simulink model "hydraulic_pilot_SimMechanics_end_US"  (R2015b)
settings: Solver=ode23t  StartTime=0.0  StopTime=1500  RelTol=1e-3
undefined symbols (not defined in the file): sigbuilder_block, X, Y, Z
libraries: sm_lib x295, fl_lib x24, nesl_utility x11, sh_lib x5, simulink x1
(part 1 of 7)
settings Model: Creator=Ivan  LastModifiedBy=Ivan
settings DataIOCC: SaveFormat=Array
settings DebuggingCC: UnderspecifiedInitializationDetection=Classic  MergeDetectMultiDrivingBlocksExec=none  SolverPrmCheckMsg=warning  StateNameClashWarn=warning
settings HardwareCC: ProdBitPerPointer=32  ProdLargestAtomicFloat=None  ProdIntDivRoundTo=Undefined  ProdEndianess=Unspecified  ProdWordSize=32  ProdHWDeviceType=32-bit Generic
settings GRTTargetCC: GeneratePreprocessorConditionals=Disable all
settings ConfigComp: CovModelRefEnable=Off
settings SimscapeCC: SimscapeLogType=all  SimscapeLogLimitData=off
settings ExplorerConfigSet: InternalSimMechanicsExplorerSettings="<ExplorerConfiguration><canonicalview>default</canonicalview><AnimationSetting><BasePlaybackSpeed>1.0</BasePlaybackSpeed><PlaybackSpeedFactor>16.0</PlaybackSpeedFactor></AnimationSetting><TilePanel><TileInfo><Tiles Columns=\"2\" Count=\"4\" Rows=\"2\"><Column Left=\"2\" Weight=\"0.5\"/><Column Left=\"554\" Weight=\"0.5\"/><Column Left=\"1106\"/><Row Top=\"2\" Weight=\"0.4992\"/><Row Top=\"320\" Weight=\"0.5008\"/><Row Top=\"639\"/><Tile Height=\"1\" Width=\"1\" X=\"0\" Y=\"0\"/><Tile Height=\"1\" Width=\"1\" X=\"0\" Y=\"1\"/><Tile Height=\"1\" Width=\"1\" X=\"1\" Y=\"0\"/><Tile Height=\"1\" Width=\"1\" X=\"1\" Y=\"1\"/></Tiles></TileInfo><SceneInfo><SceneViewer><BGColor><R>0.60000002384185791</R><G>0.60000002384185791</G><B>0.60000002384185791</B></BGColor><Camera><Position><X>-1.4545420789578025</X><Y>-0.47703526853152423</Y><Z>1.053292472596125</Z></Position><Center><X>-1.0755331343287176</X><Y>0.65681441625729753</Y><Z>0.33046154790126991</Z></Center><Up><X>0.31799715127972389</X><Y>0.43179203595848165</Y><Z>0.84405772874893448</Z></Up><Left>-0.52137946486473086</Left><Right>0.52137946486473086</Right><Bottom>-0.12744375988841058</Bottom><Top>0.12744375988841058</Top></Camera></SceneViewer><SceneViewer><BGColor><R>0.60000002384185791</R><G>0.60000002384185791</G><B>0.60000002384185791</B></BGColor><Camera><Position><X>-1.097124655307177</X><Y>0.60879350298107193</Y><Z>1.6773847746848054</Z></Position><Center><X>-1.097124655307177</X><Y>0.60879350298107193</Y><Z>0.3230140209197998</Z></Center><Up><X>0</X><Y>1</Y><Z>-0</Z></Up><Left>-0.52137946486473086</Left><Right>0.52137946486473086</Right><Bottom>-0.19162502065300943</Bottom><Top>0.19162502065300943</Top></Camera></SceneViewer><SceneViewer><BGColor><R>0.60000002384185791</R><G>0.60000002384185791</G><B>0.60000002384185791</B></BGColor><Camera><Position><X>-1.839713975613805</X><Y>1.4497817237667032</Y><Z>1.0667372871108483</Z></Position><Center><X>-1.0007040048852538</X><Y>0.55541256489420043</Y><Z>0.26430212739881542</Z></Center><Up><X>0.29701754457873719</X><Y>-0.46808723288325788</Y><Z>0.83227094183571793</Z></Up><Left>-0.47525307471029621</Left><Right>0.47525307471029621</Right><Bottom>-0.31607583672115108</Bottom><Top>0.31607583672115108</Top></Camera></SceneViewer><SceneViewer><BGColor><R>0.60000002384185791</R><G>0.60000002384185791</G><B>0.60000002384185791</B></BGColor><Camera><Position><X>-0.30663977538297038</X><Y>-0.17371608341982503</Y><Z>1.1012231263046517</Z></Position><Center><X>-1.0848488807678223</X><Y>0.60449302196502686</Y><Z>0.3230140209197998</Z></Center><Up><X>-0.40824829046386307</X><Y>0.40824829046386307</Y><Z>0.81649658092772615</Z></Up><Left>-0.50417031347751617</Left><Right>0.50417031347751617</Right><Bottom>-0.39514026045799255</Bottom><Top>0.39514026045799255</Top></Camera></SceneViewer></SceneInfo></TilePanel></ExplorerConfiguration>"

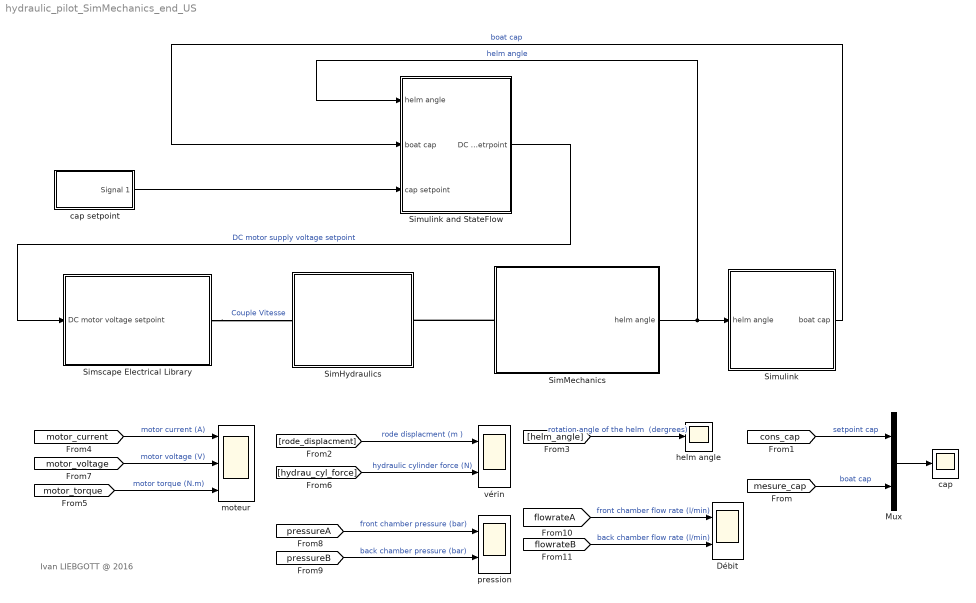
== system hydraulic_pilot_SimMechanics_end_US ==
  note: Ivan LIEBGOTT @ 2016
  " moteur" : Scope  NumInputPorts=3
  Débit : Scope  NumInputPorts=2
  Mux : Mux  Inputs=2
  SimHydraulics : Subsystem
      mask Display: image('groupe_hydraulique.jpg')
  SimMechanics : Subsystem
      mask Display: image('pilote_simmechanics.jpg')
  "Simscape Electrical Library " : Subsystem
      mask Display: image('moteur_cc_pilote.jpg')
  Simulink : Subsystem
      mask Display: image('bateau.jpg')
  Simulink and StateFlow : Subsystem
      mask Display: image('AP16_FRONT.jpg')
  "cap " : Scope
  cap setpoint : Subsystem  Tag=STV Subsys  LoadFcn=sigbuilder_block('load');  StartFcn=sigbuilder_block('start');  StopFcn=sigbuilder_block('stop');  ClipboardFcn=sigbuilder_block('clipboard');  mask(Sigbuilder block){}
      mask help: Simulink:masks:SigbuilderBlock_MD
      mask init:
      | if ~strcmp(get_param(bdroot(gcbh),'SimulationStatus'),'stopped') tuvar = sigbuilder_block('maskInit'); end
      settings: CopyFcn=sigbuilder_block('copy');  DeleteFcn=sigbuilder_block('delete');  ModelCloseFcn=sigbuilder_block('modelClose');  PreSaveFcn=sigbuilder_block('preSave');  PauseFcn=sigbuilder_block('pause');  ContinueFcn=sigbuilder_block('continue');  NameChangeFcn=sigbuilder_block('namechange');  OpenFcn=sigbuilder_block('open',[286.5 145 550.5 396 ]);  CloseFcn=sigbuilder_block('close');
      mask Display: plot(0, 0, 100, 100,[2, 2, 32, 32, 2], [68, 8, 8, 68, 68],[32, 2], [38, 38], [32, 19, 2],[53, 60, 44], [32, 17, 17, 2],[16, 16, 31, 31]);txt = getActiveGroup(gcbh);text(2, 100, txt,'verticalAlignment', 'top');
  helm angle : Scope
  pression : Scope  NumInputPorts=2
  vérin : Scope  NumInputPorts=2
  wires:
  Mux/1 -> "cap "/1
  [mesure_cap] -> Mux/2  "boat cap"
  [cons_cap] -> Mux/1  "setpoint cap"
  [rode_displacment] -> vérin/1  "rode displacment (m )"
  [helm_angle] -> helm angle/1  "rotation angle of the helm  (dergrees)"
  [motor_current] -> " moteur"/1  "motor current (A)"
  [motor_torque] -> " moteur"/3  "motor torque (N.m)"
  [hydrau_cyl_force] -> vérin/2  "hydraulic cylinder force (N)"
  cap setpoint/1(Signal 1) -> Simulink and StateFlow/3(cap setpoint)
  Simulink/1(boat cap) -> Simulink and StateFlow/2(boat cap)  "boat cap"
  Simulink and StateFlow/1(DC motor voltage setrpoint) -> "Simscape Electrical Library "/1(DC motor voltage setpoint)  "DC motor supply voltage setpoint"
  [motor_voltage] -> " moteur"/2  "motor voltage (V)"
  [pressureA] -> pression/1  "front chamber pressure (bar)"
  [pressureB] -> pression/2  "back chamber pressure (bar)"
  [flowrateA] -> Débit/1  "front chamber flow rate (l/min)"
  [flowrateB] -> Débit/2  "back chamber flow rate (l/min)"
  SimMechanics/1(helm angle) -> Simulink and StateFlow/1(helm angle), Simulink/1(helm angle)  "helm angle"
  connections:
  "Simscape Electrical Library "/RConn1 -- SimHydraulics/LConn1  "Couple Vitesse"
  SimMechanics/LConn1 -- SimHydraulics/RConn1

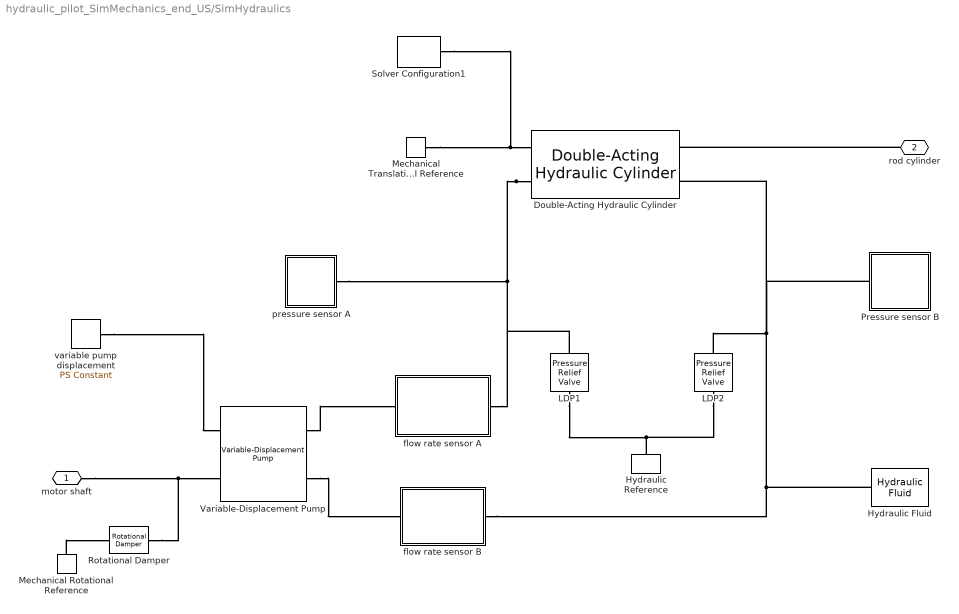
== system hydraulic_pilot_SimMechanics_end_US/SimHydraulics ==
  " LDP1" : sh_lib/Valves/Pressure Control Valves/Pressure Relief Valve  area_max=1e-4 m^2  pres_set=10e+6 Pa  reg_range=5e+5 Pa  C_d=0.7  Re_cr=12  A_leak=1e-12 m^2  dynamic=0  tau=0.1 s  area_init=1e-12 m^2  gain=1 m^2/Pa  pr_max=55e5 Pa  f_cr=100 N
  Double-Acting Hydraulic Cylinder : sh_lib/Hydraulic Cylinders/Double-Acting Hydraulic Cylinder  area_A=2e-4 m^2  area_B=2e-4 m^2  stroke=0.3 m  init_pos=0.15 m  dead_vol_A=1e-4 m^3  dead_vol_B=1e-4 m^3  init_pressure_A=0 Pa  init_pressure_B=0 Pa  k_sh=1.4  stiff=1e+6 N/m  D=150 N/(m/s)  or=1  or_sign=1
  Hydraulic Fluid : sh_lib/Hydraulic Utilities/Hydraulic Fluid  DataSource=1  SelFluid=1  SysTemp=60 c  TrapAir=0.005  ViscDerFactor=1  range_error=2
  Hydraulic Reference : fl_lib/Hydraulic/Hydraulic Elements/Hydraulic Reference
  LDP2 : sh_lib/Valves/Pressure Control Valves/Pressure Relief Valve  area_max=1e-4 m^2  pres_set=10e+6 Pa  reg_range=5e+5 Pa  C_d=0.7  Re_cr=12  A_leak=1e-12 m^2  dynamic=0  tau=0.1 s  area_init=1e-12 m^2  gain=1 m^2/Pa  pr_max=55e5 Pa  f_cr=100 N
  Mechanical Rotational Reference : fl_lib/Mechanical/Rotational Elements/Mechanical Rotational Reference
  Mechanical Translational Reference : fl_lib/Mechanical/Translational Elements/Mechanical Translational Reference
  Pressure sensor B : Subsystem
      mask Display: image('manometre.jpg')
  Rotational Damper : fl_lib/Mechanical/Rotational Elements/Rotational Damper  D=0.006 N*m/(rad/s)  w_specify=off  w_priority=None  w=0 rad/s  t_specify=off  t_priority=None  t=0 N*m
  Solver Configuration1 : nesl_utility/Solver Configuration  PhysicalDomain=network_engine_domain  SubClassName=solver  LeftPortType=input  RightPortType=generic  Accelerate=off  Tones=[]  Harmonics=[]  SimulateNoise=off  Profile=off  UseLocalSampling=off  EnableSwitchedLinearOptims=on  FrequencyDomain=off  UseCCode=off  RelTol=0.001  AbsTol=1e-06  MinStep=1e-09  ToWorkspace=off  RevertToSquareIcSolve=off  NumHomotopyIterations=100  PhasorMode=off  PhasorModeNumHarmonics=1  DoDC=off  ResidualTolerance=1e-09  UseLocalSolver=off  LocalSolverChoice=NE_BACKWARD_EULER_ADVANCER  LocalSolverSampleTime=0.001  DoFixedCost=off  MaxNonlinIter=3  MaxModeIter=2  LinearAlgebra=Sparse  DelaysMemoryBudget=1024  AutomaticFiltering=on  FilteringTimeConstant=0.001
  Variable-Displacement Pump : sh_lib/Pumps and Motors/Variable-Displacement Pump  mdl_type=1  D_max=1.77e-7 m^3/rad  stroke_max=1 m  displ_tab=[ -5e-6 -3e-6 0 3e-6 5e-6 ] m^3/rad  cntrl_mem_tab=[ -0.0075 -0.0025 0 0.0025 0.0075 ] m  interp_method=1  extrap_method=1  efficiency_vol=0.85  efficiency_tot=0.75  pr_nominal=1e+8 Pa  w_nominal=188 rad/s  visc_nominal=18 cSt  dens_nominal=900 kg/m^3  k_leak=1e-11 m^3/s/Pa  efficiency_mech=0.7
  flow rate sensor A : Subsystem
      mask Display: image('debimetre.jpg')
  flow rate sensor B : Subsystem
      mask Display: image('debimetre.jpg')
  pressure sensor A : Subsystem
      mask Display: image('manometre.jpg')
  variable pump displacement : fl_lib/Physical Signals/Sources/PS Constant  constant=0.4
  motor shaft : PMIOPort  Port=1  Side=Left
  rod cylinder : PMIOPort  Port=2  Side=Right
  connections:
  motor shaft/RConn1 -- Rotational Damper/RConn1 -- Variable-Displacement Pump/LConn2
  variable pump displacement/RConn1 -- Variable-Displacement Pump/LConn1
  rod cylinder/RConn1 -- Double-Acting Hydraulic Cylinder/RConn1
  Mechanical Translational Reference/LConn1 -- Solver Configuration1/RConn1 -- Double-Acting Hydraulic Cylinder/LConn1
  Hydraulic Fluid/RConn1 -- flow rate sensor B/RConn1 -- Pressure sensor B/LConn1 -- Double-Acting Hydraulic Cylinder/RConn2 -- LDP2/LConn1
  Hydraulic Reference/LConn1 -- " LDP1"/RConn1 -- LDP2/RConn1
  Mechanical Rotational Reference/LConn1 -- Rotational Damper/LConn1
  Double-Acting Hydraulic Cylinder/LConn2 -- flow rate sensor A/RConn1 -- " LDP1"/LConn1 -- pressure sensor A/RConn1
  Variable-Displacement Pump/RConn1 -- flow rate sensor A/LConn1
  Variable-Displacement Pump/RConn2 -- flow rate sensor B/LConn1

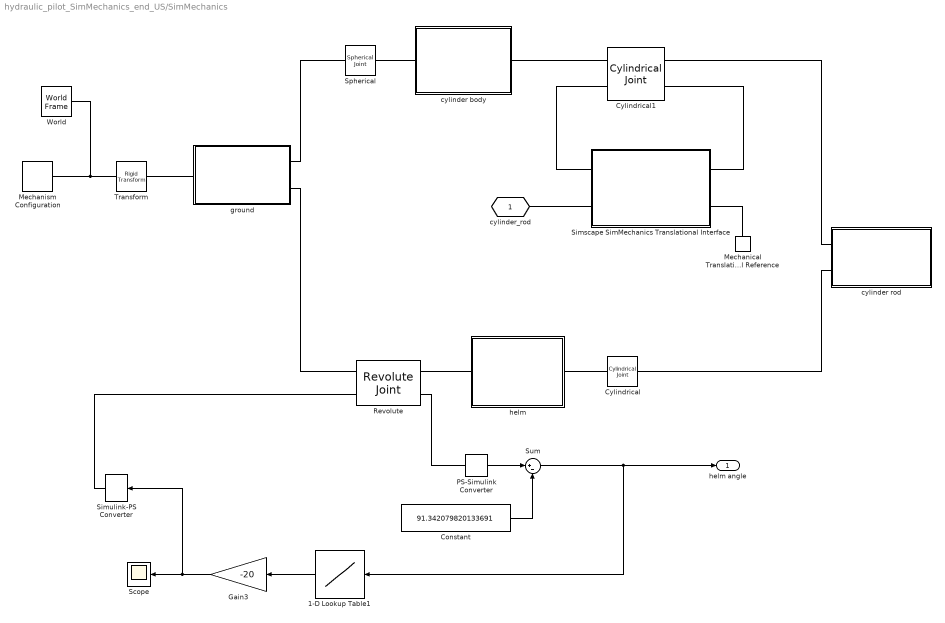
== system hydraulic_pilot_SimMechanics_end_US/SimMechanics ==
  1-D Lookup Table1 : Lookup_n-D  NumberOfTableDimensions=1  BreakpointsForDimension1=[0 5 10 15 20 25 30]  Table=[0 2.5 5 10 30 60 100]  RndMeth=Simplest  InputSameDT=on
  Constant : Constant  Value=91.342079820133691
  Cylindrical : sm_lib/Joints/Cylindrical Joint  SenseConstraintForce=off  SenseConstraintForceX=off  SenseConstraintForceY=off  SenseConstraintForceZ=off  SenseConstraintTorque=off  SenseConstraintTorqueX=off  SenseConstraintTorqueY=off  SenseConstraintTorqueZ=off  SenseTotalForce=off  SenseTotalForceX=off  SenseTotalForceY=off  SenseTotalForceZ=off  SenseTotalTorque=off  SenseTotalTorqueX=off  SenseTotalTorqueY=off  SenseTotalTorqueZ=off  CompositeWrenchDir=FollowerOnBase  CompositeWrenchFrame=BaseFrame  PzEquilibriumPosition=0  PzEquilibriumPositionUnits=m  PzSpringStiffness=0  PzSpringStiffnessUnits=N/m  PzDampingCoefficient=0  PzDampingCoefficientUnits=s*N/m  PzTorqueActuationMode=NoTorque  PzMotionActuationMode=ComputedMotion  PzSensePosition=off  PzSenseVelocity=off  PzSenseAcceleration=off  PzSenseTorqueForce=off  PzPositionTargetSpecify=on  PzPositionTargetPriority=Low  PzPositionTargetValue=0  PzPositionTargetValueUnits=m  PzVelocityTargetSpecify=off  PzVelocityTargetPriority=High  PzVelocityTargetValue=0  PzVelocityTargetValueUnits=m/s  RzEquilibriumPosition=0  RzEquilibriumPositionUnits=rad  RzSpringStiffness=0  RzSpringStiffnessUnits=m*N/rad  RzDampingCoefficient=0  RzDampingCoefficientUnits=m*s*N/rad  RzTorqueActuationMode=NoTorque  RzMotionActuationMode=ComputedMotion  RzSensePosition=off  RzSenseVelocity=off  RzSenseAcceleration=off  RzSenseTorqueForce=off  RzPositionTargetSpecify=on  RzPositionTargetPriority=Low  RzPositionTargetValue=88.917590363493801  RzPositionTargetValueUnits=deg  RzVelocityTargetSpecify=off  RzVelocityTargetPriority=High  RzVelocityTargetValue=0  RzVelocityTargetValueUnits=deg/s  BlockFunction=simmechanics.library.joints.cylindrical_joint
  Cylindrical1 : sm_lib/Joints/Cylindrical Joint  SenseConstraintForce=off  SenseConstraintForceX=off  SenseConstraintForceY=off  SenseConstraintForceZ=off  SenseConstraintTorque=off  SenseConstraintTorqueX=off  SenseConstraintTorqueY=off  SenseConstraintTorqueZ=off  SenseTotalForce=off  SenseTotalForceX=off  SenseTotalForceY=off  SenseTotalForceZ=off  SenseTotalTorque=off  SenseTotalTorqueX=off  SenseTotalTorqueY=off  SenseTotalTorqueZ=off  CompositeWrenchDir=FollowerOnBase  CompositeWrenchFrame=BaseFrame  PzEquilibriumPosition=0  PzEquilibriumPositionUnits=m  PzSpringStiffness=0  PzSpringStiffnessUnits=N/m  PzDampingCoefficient=200  PzDampingCoefficientUnits=s*N/m  PzTorqueActuationMode=InputTorque  PzMotionActuationMode=ComputedMotion  PzSensePosition=off  PzSenseVelocity=on  PzSenseAcceleration=off  PzSenseTorqueForce=off  PzPositionTargetSpecify=on  PzPositionTargetPriority=Low  PzPositionTargetValue=0  PzPositionTargetValueUnits=m  PzVelocityTargetSpecify=off  PzVelocityTargetPriority=High  PzVelocityTargetValue=0  PzVelocityTargetValueUnits=m/s  RzEquilibriumPosition=0  RzEquilibriumPositionUnits=rad  RzSpringStiffness=0  RzSpringStiffnessUnits=m*N/rad  RzDampingCoefficient=1  RzDampingCoefficientUnits=m*s*N/rad  RzTorqueActuationMode=NoTorque  RzMotionActuationMode=ComputedMotion  RzSensePosition=off  RzSenseVelocity=off  RzSenseAcceleration=off  RzSenseTorqueForce=off  RzPositionTargetSpecify=on  RzPositionTargetPriority=Low  RzPositionTargetValue=-151.66852375213551  RzPositionTargetValueUnits=deg  RzVelocityTargetSpecify=off  RzVelocityTargetPriority=High  RzVelocityTargetValue=0  RzVelocityTargetValueUnits=deg/s  BlockFunction=simmechanics.library.joints.cylindrical_joint
  Gain3 : Gain  Gain=-20
  Mechanical Translational Reference : fl_lib/Mechanical/Translational Elements/Mechanical Translational Reference
  Mechanism Configuration : sm_lib/Utilities/Mechanism Configuration  UniformGravity=Constant  GravityVector=[0 0 -9.81]  GravityUnits=m/s^2  LinearizationDelta=0.001  BlockFunction=simmechanics.library.utilities.mechanism_configuration
  PS-Simulink Converter : nesl_utility/PS-Simulink Converter  PhysicalDomain=network_engine_domain  SubClassName=ps_output  LeftPortType=input  RightPortType=output  PseudoPeriodic=off  Frequencies=[]  Unit=deg  AffineConversion=off
  Revolute : sm_lib/Joints/Revolute Joint  SenseConstraintForce=off  SenseConstraintForceX=off  SenseConstraintForceY=off  SenseConstraintForceZ=off  SenseConstraintTorque=off  SenseConstraintTorqueX=off  SenseConstraintTorqueY=off  SenseConstraintTorqueZ=off  SenseTotalForce=off  SenseTotalForceX=off  SenseTotalForceY=off  SenseTotalForceZ=off  SenseTotalTorque=off  SenseTotalTorqueX=off  SenseTotalTorqueY=off  SenseTotalTorqueZ=off  CompositeWrenchDir=FollowerOnBase  CompositeWrenchFrame=BaseFrame  EquilibriumPosition=0  EquilibriumPositionUnits=rad  SpringStiffness=0  SpringStiffnessUnits=m*N/rad  DampingCoefficient=0  DampingCoefficientUnits=m*s*N/rad  TorqueActuationMode=InputTorque  MotionActuationMode=ComputedMotion  SensePosition=on  SenseVelocity=off  SenseAcceleration=off  SenseTorqueForce=off  PositionTargetSpecify=on  PositionTargetPriority=Low  PositionTargetValue=91.342079820133691  PositionTargetValueUnits=deg  VelocityTargetSpecify=off  VelocityTargetPriority=High  VelocityTargetValue=0  VelocityTargetValueUnits=deg/s  BlockFunction=simmechanics.library.joints.revolute_joint
  Scope : Scope
  Simscape SimMechanics Translational Interface : Subsystem
  Simulink-PS Converter : nesl_utility/Simulink-PS Converter  PhysicalDomain=network_engine_domain  SubClassName=ps_input  LeftPortType=input  RightPortType=output  PseudoPeriodic=off  Frequencies=[]  NoiseDistribution=none  NoiseParameters=[]  Unit=1  AffineConversion=off  InputFiltering=off  SimscapeFilterOrder=1  InputFilterTimeConstant=0.001  UdotUserProvided=1
  Spherical : sm_lib/Joints/Spherical Joint  SenseConstraintForce=off  SenseConstraintForceX=off  SenseConstraintForceY=off  SenseConstraintForceZ=off  SenseConstraintTorque=off  SenseConstraintTorqueX=off  SenseConstraintTorqueY=off  SenseConstraintTorqueZ=off  SenseTotalForce=off  SenseTotalForceX=off  SenseTotalForceY=off  SenseTotalForceZ=off  SenseTotalTorque=off  SenseTotalTorqueX=off  SenseTotalTorqueY=off  SenseTotalTorqueZ=off  CompositeWrenchDir=FollowerOnBase  CompositeWrenchFrame=BaseFrame  DefPosRotationMethod=None  DefPosRotationAngleUnits=deg  DefPosRotationStandardAxis=+Z  DefPosRotationAngle=0  DefPosRotationArbitraryAxis=[0 0 1]  DefPosFollAlignAxisA=+X  DefPosBaseAlignAxisA=+Y  DefPosFollAlignAxisB=+Y  DefPosBaseAlignAxisB=+Z  DefPosRotationSequenceAxes=FollowerAxes  DefPosRotationSequence=XYX  DefPosRotationSequenceAngles=[0 0 0]  DefPosRotationSequenceAnglesUnits=deg  DefPosRotationMatrix=[1 0 0; 0 1 0; 0 0 1]  EqPosRotationMethod=None  EqPosRotationAngleUnits=deg  EqPosRotationStandardAxis=+Z  EqPosRotationAngle=0  EqPosRotationArbitraryAxis=[0 0 1]  EqPosFollAlignAxisA=+X  EqPosBaseAlignAxisA=+Y  EqPosFollAlignAxisB=+Y  EqPosBaseAlignAxisB=+Z  EqPosRotationSequenceAxes=FollowerAxes  EqPosRotationSequence=XYX  EqPosRotationSequenceAngles=[0 0 0]  EqPosRotationSequenceAnglesUnits=deg  EqPosRotationMatrix=[1 0 0; 0 1 0; 0 0 1]  SpringStiffness=0  SpringStiffnessUnits=m*N/rad  DampingCoefficient=0  DampingCoefficientUnits=m*s*N/rad  ActuateTorqueX=off  ActuateTorqueY=off  ActuateTorqueZ=off  ActuateTorque=off  TorqueActuationMode=NoTorque  MotionActuationMode=ComputedMotion  ActuationFrame=BaseFrame  SensePosition=off  SenseVelocityX=off  SenseVelocityY=off  SenseVelocityZ=off  SenseVelocity=off  SenseAccelerationX=off  SenseAccelerationY=off  SenseAccelerationZ=off  SenseAcceleration=off  SenseTorqueX=off  SenseTorqueY=off  SenseTorqueZ=off  SenseTorqueForce=off  SensingFrame=FollowerFrame  PositionTargetRotationMethod=None  PositionTargetRotationAngleUnits=deg  PositionTargetRotationStandardAxis=+Z  PositionTargetRotationAngle=0  PositionTargetRotationArbitraryAxis=[0 0 1]  PositionTargetFollAlignAxisA=+X  PositionTargetBaseAlignAxisA=+Y  PositionTargetFollAlignAxisB=+Y  PositionTargetBaseAlignAxisB=+Z  PositionTargetRotationSequenceAxes=FollowerAxes  PositionTargetRotationSequence=XYX  PositionTargetRotationSequenceAngles=[0 0 0]  PositionTargetRotationSequenceAnglesUnits=deg  PositionTargetRotationMatrix=[1 0 0; 0 1 0; 0 0 1]  PositionTargetSpecify=off  PositionTargetPriority=High  VelocityTargetValue=[0 0 0]  VelocityTargetValueUnits=deg/s  VelocityTargetSpecify=off  VelocityTargetPriority=High  VelocityTargetInFollowerFrame=on  BlockFunction=simmechanics.library.joints.spherical_joint
  Sum : Sum  Inputs=|+-
  Transform : sm_lib/Frames and Transforms/Rigid Transform  TranslationMethod=Cartesian  TranslationLengthUnit=mm  TranslationStandardAxis=+Z  TranslationStandardOffset=0  TranslationCartesianOffset=[-854.29700000000003 517.99300000000005 336.38900000000001]  TranslationROffset=0  TranslationROffsetUnits=m  TranslationZOffset=0  TranslationZOffsetUnits=m  TranslationThetaOffset=0  TranslationThetaOffsetUnits=deg  RotationMethod=None  RotationAngleUnits=deg  RotationStandardAxis=+Z  RotationAngle=0  RotationArbitraryAxis=[0 0 1]  FollAlignAxisA=+X  BaseAlignAxisA=+Y  FollAlignAxisB=+Y  BaseAlignAxisB=+Z  RotationSequenceAxes=FollowerAxes  RotationSequence=XYX  RotationSequenceAngles=[0 0 0]  RotationSequenceAnglesUnits=deg  RotationMatrix=[1 0 0; 0 1 0; 0 0 1]  BlockFunction=simmechanics.library.frames_transforms.rigid_transform
  World : sm_lib/Frames and Transforms/World Frame  BlockFunction=simmechanics.library.frames_transforms.world_frame
  cylinder body : Subsystem
      mask Display: image('cylindre.jpg')
  cylinder rod : Subsystem
      mask Display: image('tige1.jpg')
  ground : Subsystem
      mask Display: image('bati1.jpg')
  helm : Subsystem
      mask Display: image('meche.jpg')
  "cylinder_rod " : PMIOPort  Port=1  Side=Left
  helm angle : Outport
  wires:
  Constant/1 -> Sum/2
  Sum/1 -> 1-D Lookup Table1/1, helm angle/1
  1-D Lookup Table1/1 -> Gain3/1
  Gain3/1 -> Simulink-PS Converter/1, Scope/1
  PS-Simulink Converter/1 -> Sum/1
  connections:
  World/RConn1 -- Transform/LConn1 -- Mechanism Configuration/RConn1
  Revolute/RConn1 -- helm/LConn1
  cylinder body/LConn1 -- Spherical/RConn1
  Cylindrical1/RConn1 -- cylinder rod/LConn1
  Cylindrical/LConn1 -- helm/RConn1
  Cylindrical/RConn1 -- cylinder rod/LConn2
  ground/RConn1 -- Spherical/LConn1
  ground/LConn1 -- Transform/RConn1
  Revolute/LConn1 -- ground/RConn2
  Cylindrical1/LConn1 -- cylinder body/RConn1
  Cylindrical1/RConn2 -- Simscape SimMechanics Translational Interface/RConn1
  Mechanical Translational Reference/LConn1 -- Simscape SimMechanics Translational Interface/RConn2
  "cylinder_rod "/RConn1 -- Simscape SimMechanics Translational Interface/LConn2
  Simscape SimMechanics Translational Interface/LConn1 -- Cylindrical1/LConn2
  Revolute/RConn2 -- PS-Simulink Converter/LConn1
  Simulink-PS Converter/RConn1 -- Revolute/LConn2

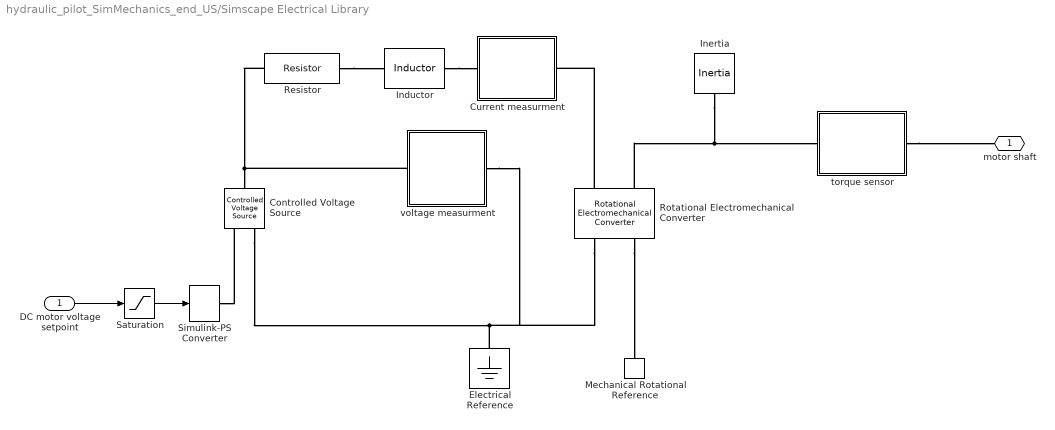
== system hydraulic_pilot_SimMechanics_end_US/Simscape Electrical Library  ==
  DC motor voltage setpoint : Inport
  Controlled Voltage Source : fl_lib/Electrical/Electrical Sources/Controlled Voltage Source
  Current measurment : Subsystem
      mask Display: image('ampermetre.jpg')
  Electrical Reference : fl_lib/Electrical/Electrical Elements/Electrical Reference
  Inductor : fl_lib/Electrical/Electrical Elements/Inductor  l=1e-7 H  r=0 Ohm  g=1e-9 1/Ohm  i_specify=off  i_priority=None  i=0 A  v_specify=off  v_priority=None  v=0 V  i_L_specify=on  i_L_priority=High  i_L=0 A
  Inertia : fl_lib/Mechanical/Rotational Elements/Inertia  inertia=0.005 kg*m^2  w_specify=on  w_priority=High  w=0 rad/s  t_specify=off  t_priority=None  t=0 N*m
  Mechanical Rotational Reference : fl_lib/Mechanical/Rotational Elements/Mechanical Rotational Reference
  Resistor : fl_lib/Electrical/Electrical Elements/Resistor  R=0.247 Ohm  i_specify=off  i_priority=None  i=0 A  v_specify=off  v_priority=None  v=0 V
  Rotational Electromechanical Converter : fl_lib/Electrical/Electrical Elements/Rotational Electromechanical Converter  K=0.047 V/(rad/s)  i_specify=off  i_priority=None  i=0 A  v_specify=off  v_priority=None  v=0 V  t_specify=off  t_priority=None  t=0 N*m  w_specify=off  w_priority=None  w=0 rad/s
  Saturation : Saturate  UpperLimit=12  LowerLimit=-12
  Simulink-PS Converter : nesl_utility/Simulink-PS Converter  PhysicalDomain=network_engine_domain  SubClassName=ps_input  LeftPortType=input  RightPortType=output  PseudoPeriodic=off  Frequencies=[]  NoiseDistribution=none  NoiseParameters=[]  Unit=V  AffineConversion=off  InputFiltering=off  SimscapeFilterOrder=1  InputFilterTimeConstant=0.001  UdotUserProvided=1
  torque sensor : Subsystem
      mask Display: image('couplemetre.jpg')
  voltage measurment : Subsystem
      mask Display: image('voltmetre.jpg')
  motor shaft : PMIOPort  Port=1  Side=Right
  wires:
  DC motor voltage setpoint/1 -> Saturation/1
  Saturation/1 -> Simulink-PS Converter/1
  connections:
  Simulink-PS Converter/RConn1 -- Controlled Voltage Source/RConn1
  Rotational Electromechanical Converter/RConn2 -- Mechanical Rotational Reference/LConn1
  Electrical Reference/LConn1 -- Controlled Voltage Source/RConn2 -- voltage measurment/RConn1 -- Rotational Electromechanical Converter/RConn1
  Resistor/LConn1 -- voltage measurment/LConn1 -- Controlled Voltage Source/LConn1
  Resistor/RConn1 -- Inductor/LConn1
  Inductor/RConn1 -- Current measurment/LConn1
  Rotational Electromechanical Converter/LConn1 -- Current measurment/RConn1
  Inertia/LConn1 -- Rotational Electromechanical Converter/LConn2 -- torque sensor/LConn1
  torque sensor/RConn1 -- motor shaft/RConn1

== system hydraulic_pilot_SimMechanics_end_US/Simulink ==
  helm angle : Inport
  Integrator : Integrator
  Perturbation : Subsystem
      mask Display: image('vague.jpg')
  Sum : Sum  Inputs=-+|
  Transfer Fcn1 : TransferFcn  Numerator=[0.005]  Denominator=[1 0.1]
  boat cap : Outport
  wires:
  helm angle/1 -> Transfer Fcn1/1
  Integrator/1 -> boat cap/1
  Sum/1 -> Integrator/1
  Transfer Fcn1/1 -> Sum/2
  Perturbation/1(Out1) -> Sum/1

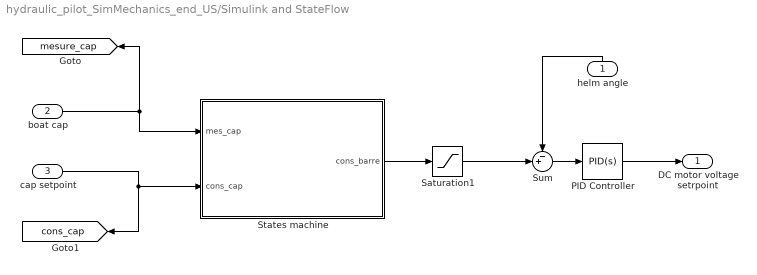
== system hydraulic_pilot_SimMechanics_end_US/Simulink and StateFlow ==
  helm angle : Inport
  boat cap : Inport  Port=2
  cap setpoint : Inport  Port=3
  PID Controller : simulink/Continuous/PID Controller  Controller=PID  TimeDomain=Continuous-time  SampleTime=-1  IntegratorMethod=Forward Euler  FilterMethod=Forward Euler  Form=Parallel  UseFilter=on  ControllerParametersSource=internal  P=0.5  I=0.001  D=0  N=100  InitialConditionSource=internal  InitialConditionForIntegrator=0  InitialConditionForFilter=0  ExternalReset=none  LimitOutput=off  UpperSaturationLimit=inf  LowerSaturationLimit=-inf  LinearizeAsGain=on  AntiWindupMode=none  Kb=1  TrackingMode=off  Kt=1  PParamMin=[]  PParamMax=[]  IParamMin=[]  IParamMax=[]  DParamMin=[]  DParamMax=[]  NParamMin=[]  NParamMax=[]  KbParamMin=[]  KbParamMax=[]  KtParamMin=[]  KtParamMax=[]  POutMin=[]  POutMax=[]  IOutMin=[]  IOutMax=[]  DOutMin=[]  DOutMax=[]  NOutMin=[]  NOutMax=[]  KbOutMin=[]  KbOutMax=[]  KtOutMin=[]  KtOutMax=[]  IntegratorOutMin=[]  IntegratorOutMax=[]  FilterOutMin=[]  FilterOutMax=[]  SumOutMin=[]  SumOutMax=[]  SumI1OutMin=[]  SumI1OutMax=[]  SumI2OutMin=[]  SumI2OutMax=[]  SumI3OutMin=[]  SumI3OutMax=[]  SumDOutMin=[]  SumDOutMax=[]  SaturationOutMin=[]  SaturationOutMax=[]  IntegratorContinuousStateAttributes=''  IntegratorStateMustResolveToSignalObject=off  IntegratorRTWStateStorageClass=Auto  FilterContinuousStateAttributes=''  FilterStateMustResolveToSignalObject=off  FilterRTWStateStorageClass=Auto  DifferentiatorICPrevScaledInput=0  DifferentiatorOutMin=[]  DifferentiatorOutMax=[]
  Saturation1 : Saturate  UpperLimit=25  LowerLimit=-25
  States machine : Stateflow chart  TreatAsAtomicUnit=on
  Sum : Sum  Inputs=-+|
  DC motor voltage setrpoint : Outport
  tag scope: cons_cap=global, mesure_cap=global
  wires:
  helm angle/1 -> Sum/1
  cap setpoint/1 -> States machine/2(cons_cap), [cons_cap]
  boat cap/1 -> [mesure_cap], States machine/1(mes_cap)
  Sum/1 -> PID Controller/1
  PID Controller/1 -> DC motor voltage setrpoint/1
  States machine/1(cons_barre) -> Saturation1/1
  Saturation1/1 -> Sum/2

== system hydraulic_pilot_SimMechanics_end_US/cap setpoint ==
  Demux : Demux  Tag=STV Demux  Outputs=1
  FromWs : FromWorkspace  Tag=STV FromWs  VariableName=tuvar  SampleTime=0
      SigBuilderData=|
      | common.afterFinalStr = 'Extrapolate'
      | common.sampleTime = 0
      | dataSet.timeRange = [0 1500]
      | dataSet.name = 'Group 1'
      | sbobj.Groups.Name = 'Group 1'
      | sbobj.Groups.Signals.Name = 'Signal 1'
      | sbobj.Groups.Signals.XData = [0 502 502 1500]
      | sbobj.Groups.Signals.YData = [20 20 -40 -40]
      | sbobj.Groups.TimeRange = [0 1500]
  Signal 1 : Outport  Tag=STV Outport
  wires:
  Demux/1 -> Signal 1/1
  FromWs/1 -> Demux/1

== system hydraulic_pilot_SimMechanics_end_US/SimHydraulics/Pressure sensor B ==
  Hydraulic Pressure Sensor1 : fl_lib/Hydraulic/Hydraulic Sensors/Hydraulic Pressure Sensor
  Hydraulic Reference2 : fl_lib/Hydraulic/Hydraulic Elements/Hydraulic Reference
  PS-Simulink Converter3 : nesl_utility/PS-Simulink Converter  PhysicalDomain=network_engine_domain  SubClassName=ps_output  LeftPortType=input  RightPortType=output  PseudoPeriodic=off  Frequencies=[]  Unit=bar  AffineConversion=off
  Conn1 : PMIOPort  Port=1  Side=Left
  tag scope: pressureB=global
  wires:
  PS-Simulink Converter3/1 -> [pressureB]
  connections:
  Hydraulic Reference2/LConn1 -- Hydraulic Pressure Sensor1/RConn1
  Hydraulic Pressure Sensor1/RConn2 -- PS-Simulink Converter3/LConn1
  Hydraulic Pressure Sensor1/LConn1 -- Conn1/RConn1

== system hydraulic_pilot_SimMechanics_end_US/SimHydraulics/flow rate sensor A ==
  Hydraulic Flow Rate Sensor : fl_lib/Hydraulic/Hydraulic Sensors/Hydraulic Flow Rate Sensor
  PS-Simulink Converter4 : nesl_utility/PS-Simulink Converter  PhysicalDomain=network_engine_domain  SubClassName=ps_output  LeftPortType=input  RightPortType=output  PseudoPeriodic=off  Frequencies=[]  Unit=l/min  AffineConversion=off
  Conn1 : PMIOPort  Port=1  Side=Right
  Conn2 : PMIOPort  Port=2  Side=Left
  tag scope: flowrateA=global
  wires:
  PS-Simulink Converter4/1 -> [flowrateA]
  connections:
  Conn2/RConn1 -- Hydraulic Flow Rate Sensor/LConn1
  Hydraulic Flow Rate Sensor/RConn1 -- PS-Simulink Converter4/LConn1
  Hydraulic Flow Rate Sensor/RConn2 -- Conn1/RConn1

== system hydraulic_pilot_SimMechanics_end_US/SimHydraulics/flow rate sensor B ==
  Hydraulic Flow Rate Sensor1 : fl_lib/Hydraulic/Hydraulic Sensors/Hydraulic Flow Rate Sensor
  PS-Simulink Converter5 : nesl_utility/PS-Simulink Converter  PhysicalDomain=network_engine_domain  SubClassName=ps_output  LeftPortType=input  RightPortType=output  PseudoPeriodic=off  Frequencies=[]  Unit=l/min  AffineConversion=off
  Conn1 : PMIOPort  Port=1  Side=Right
  Conn2 : PMIOPort  Port=2  Side=Left
  tag scope: flowrateB=global
  wires:
  PS-Simulink Converter5/1 -> [flowrateB]
  connections:
  Conn2/RConn1 -- Hydraulic Flow Rate Sensor1/LConn1
  Hydraulic Flow Rate Sensor1/RConn1 -- PS-Simulink Converter5/LConn1
  Hydraulic Flow Rate Sensor1/RConn2 -- Conn1/RConn1

== system hydraulic_pilot_SimMechanics_end_US/SimHydraulics/pressure sensor A ==
  Hydraulic Pressure Sensor : fl_lib/Hydraulic/Hydraulic Sensors/Hydraulic Pressure Sensor
  Hydraulic Reference1 : fl_lib/Hydraulic/Hydraulic Elements/Hydraulic Reference
  PS-Simulink Converter2 : nesl_utility/PS-Simulink Converter  PhysicalDomain=network_engine_domain  SubClassName=ps_output  LeftPortType=input  RightPortType=output  PseudoPeriodic=off  Frequencies=[]  Unit=bar  AffineConversion=off
  Conn1 : PMIOPort  Port=1  Side=Right
  tag scope: pressureA=global
  wires:
  PS-Simulink Converter2/1 -> [pressureA]
  connections:
  Hydraulic Pressure Sensor/LConn1 -- Conn1/RConn1
  PS-Simulink Converter2/LConn1 -- Hydraulic Pressure Sensor/RConn2
  Hydraulic Reference1/LConn1 -- Hydraulic Pressure Sensor/RConn1

== system hydraulic_pilot_SimMechanics_end_US/SimMechanics/Simscape SimMechanics Translational Interface ==
  Ideal Force Sensor1 : fl_lib/Mechanical/Mechanical Sensors/Ideal Force Sensor
  Ideal Translational Velocity Source1 : fl_lib/Mechanical/Mechanical Sources/Ideal Translational Velocity Source
  actuation force : PMIOPort  Port=1  Side=Left
  velocity feedback : PMIOPort  Port=2  Side=Right
  Simscape input : PMIOPort  Port=3  Side=Left
  velocity reference : PMIOPort  Port=4  Side=Right
  connections:
  Ideal Force Sensor1/RConn2 -- actuation force/RConn1
  Ideal Force Sensor1/LConn1 -- Simscape input/RConn1
  Ideal Translational Velocity Source1/RConn2 -- velocity reference/RConn1
  Ideal Translational Velocity Source1/LConn1 -- Ideal Force Sensor1/RConn1
  velocity feedback/RConn1 -- Ideal Translational Velocity Source1/RConn1

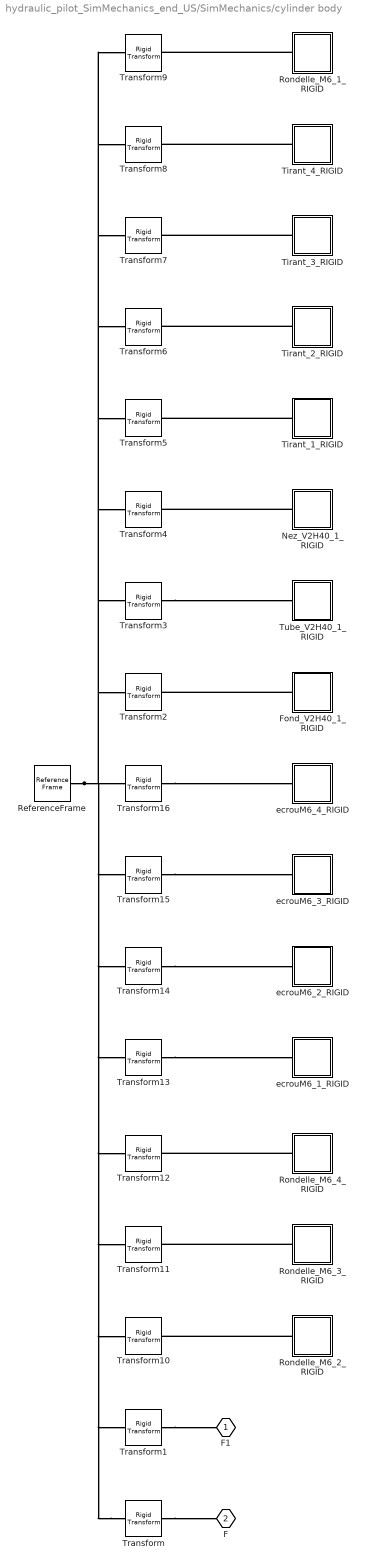
== system hydraulic_pilot_SimMechanics_end_US/SimMechanics/cylinder body ==
  Fond_V2H40_1_RIGID : Subsystem
  Nez_V2H40_1_RIGID : Subsystem
  ReferenceFrame : sm_lib/Frames and Transforms/Reference Frame  BlockFunction=simmechanics.library.frames_transforms.reference_frame
  Rondelle_M6_1_RIGID : Subsystem
  Rondelle_M6_2_RIGID : Subsystem
  Rondelle_M6_3_RIGID : Subsystem
  Rondelle_M6_4_RIGID : Subsystem
  Tirant_1_RIGID : Subsystem
  Tirant_2_RIGID : Subsystem
  Tirant_3_RIGID : Subsystem
  Tirant_4_RIGID : Subsystem
  Transform : sm_lib/Frames and Transforms/Rigid Transform  TranslationMethod=Cartesian  TranslationLengthUnit=mm  TranslationStandardAxis=+Z  TranslationStandardOffset=0  TranslationCartesianOffset=[188.721 92.663199999999904 -65.118999999999957]  TranslationROffset=0  TranslationROffsetUnits=m  TranslationZOffset=0  TranslationZOffsetUnits=m  TranslationThetaOffset=0  TranslationThetaOffsetUnits=deg  RotationMethod=ArbitraryAxis  RotationAngleUnits=rad  RotationStandardAxis=+Z  RotationAngle=2.0943951023931957  RotationArbitraryAxis=[-0.57735026918962584 -0.57735026918962573 0.57735026918962573]  FollAlignAxisA=+X  BaseAlignAxisA=+Y  FollAlignAxisB=+Y  BaseAlignAxisB=+Z  RotationSequenceAxes=FollowerAxes  RotationSequence=XYX  RotationSequenceAngles=[0 0 0]  RotationSequenceAnglesUnits=deg  RotationMatrix=[1 0 0; 0 1 0; 0 0 1]  BlockFunction=simmechanics.library.frames_transforms.rigid_transform
  Transform1 : sm_lib/Frames and Transforms/Rigid Transform  TranslationMethod=Cartesian  TranslationLengthUnit=mm  TranslationStandardAxis=+Z  TranslationStandardOffset=0  TranslationCartesianOffset=[-156.47941139923006 92.663279084864655 -65.118488806106384]  TranslationROffset=0  TranslationROffsetUnits=m  TranslationZOffset=0  TranslationZOffsetUnits=m  TranslationThetaOffset=0  TranslationThetaOffsetUnits=deg  RotationMethod=ArbitraryAxis  RotationAngleUnits=rad  RotationStandardAxis=+Z  RotationAngle=0  RotationArbitraryAxis=[0 0 0]  FollAlignAxisA=+X  BaseAlignAxisA=+Y  FollAlignAxisB=+Y  BaseAlignAxisB=+Z  RotationSequenceAxes=FollowerAxes  RotationSequence=XYX  RotationSequenceAngles=[0 0 0]  RotationSequenceAnglesUnits=deg  RotationMatrix=[1 0 0; 0 1 0; 0 0 1]  BlockFunction=simmechanics.library.frames_transforms.rigid_transform
  Transform10 : sm_lib/Frames and Transforms/Rigid Transform  TranslationMethod=Cartesian  TranslationLengthUnit=mm  TranslationStandardAxis=+Z  TranslationStandardOffset=0  TranslationCartesianOffset=[-113.27900000000001 82.1584 -39.164299999999997]  TranslationROffset=0  TranslationROffsetUnits=m  TranslationZOffset=0  TranslationZOffsetUnits=m  TranslationThetaOffset=0  TranslationThetaOffsetUnits=deg  RotationMethod=ArbitraryAxis  RotationAngleUnits=rad  RotationStandardAxis=+Z  RotationAngle=1.6089415653150072  RotationArbitraryAxis=[0.19166392654548026 -0.96256422046652934 -0.19166392654548026]  FollAlignAxisA=+X  BaseAlignAxisA=+Y  FollAlignAxisB=+Y  BaseAlignAxisB=+Z  RotationSequenceAxes=FollowerAxes  RotationSequence=XYX  RotationSequenceAngles=[0 0 0]  RotationSequenceAnglesUnits=deg  RotationMatrix=[1 0 0; 0 1 0; 0 0 1]  BlockFunction=simmechanics.library.frames_transforms.rigid_transform
  Transform11 : sm_lib/Frames and Transforms/Rigid Transform  TranslationMethod=Cartesian  TranslationLengthUnit=mm  TranslationStandardAxis=+Z  TranslationStandardOffset=0  TranslationCartesianOffset=[-113.27900000000001 66.708399999999997 -75.623800000000003]  TranslationROffset=0  TranslationROffsetUnits=m  TranslationZOffset=0  TranslationZOffsetUnits=m  TranslationThetaOffset=0  TranslationThetaOffsetUnits=deg  RotationMethod=ArbitraryAxis  RotationAngleUnits=rad  RotationStandardAxis=+Z  RotationAngle=1.6089415653150072  RotationArbitraryAxis=[0.19166392654548026 -0.96256422046652934 -0.19166392654548026]  FollAlignAxisA=+X  BaseAlignAxisA=+Y  FollAlignAxisB=+Y  BaseAlignAxisB=+Z  RotationSequenceAxes=FollowerAxes  RotationSequence=XYX  RotationSequenceAngles=[0 0 0]  RotationSequenceAnglesUnits=deg  RotationMatrix=[1 0 0; 0 1 0; 0 0 1]  BlockFunction=simmechanics.library.frames_transforms.rigid_transform
  Transform12 : sm_lib/Frames and Transforms/Rigid Transform  TranslationMethod=Cartesian  TranslationLengthUnit=mm  TranslationStandardAxis=+Z  TranslationStandardOffset=0  TranslationCartesianOffset=[-113.27900000000001 103.16799999999999 -91.073799999999991]  TranslationROffset=0  TranslationROffsetUnits=m  TranslationZOffset=0  TranslationZOffsetUnits=m  TranslationThetaOffset=0  TranslationThetaOffsetUnits=deg  RotationMethod=ArbitraryAxis  RotationAngleUnits=rad  RotationStandardAxis=+Z  RotationAngle=1.6089415653150072  RotationArbitraryAxis=[0.19166392654548026 -0.96256422046652934 -0.19166392654548026]  FollAlignAxisA=+X  BaseAlignAxisA=+Y  FollAlignAxisB=+Y  BaseAlignAxisB=+Z  RotationSequenceAxes=FollowerAxes  RotationSequence=XYX  RotationSequenceAngles=[0 0 0]  RotationSequenceAnglesUnits=deg  RotationMatrix=[1 0 0; 0 1 0; 0 0 1]  BlockFunction=simmechanics.library.frames_transforms.rigid_transform
  Transform13 : sm_lib/Frames and Transforms/Rigid Transform  TranslationMethod=Cartesian  TranslationLengthUnit=mm  TranslationStandardAxis=+Z  TranslationStandardOffset=0  TranslationCartesianOffset=[-119.67899999999999 103.16799999999999 -91.073799999999991]  TranslationROffset=0  TranslationROffsetUnits=m  TranslationZOffset=0  TranslationZOffsetUnits=m  TranslationThetaOffset=0  TranslationThetaOffsetUnits=deg  RotationMethod=ArbitraryAxis  RotationAngleUnits=rad  RotationStandardAxis=+Z  RotationAngle=1.5707963267948968  RotationArbitraryAxis=[0 1 0]  FollAlignAxisA=+X  BaseAlignAxisA=+Y  FollAlignAxisB=+Y  BaseAlignAxisB=+Z  RotationSequenceAxes=FollowerAxes  RotationSequence=XYX  RotationSequenceAngles=[0 0 0]  RotationSequenceAnglesUnits=deg  RotationMatrix=[1 0 0; 0 1 0; 0 0 1]  BlockFunction=simmechanics.library.frames_transforms.rigid_transform
  Transform14 : sm_lib/Frames and Transforms/Rigid Transform  TranslationMethod=Cartesian  TranslationLengthUnit=mm  TranslationStandardAxis=+Z  TranslationStandardOffset=0  TranslationCartesianOffset=[-119.67899999999999 66.708399999999997 -75.623800000000003]  TranslationROffset=0  TranslationROffsetUnits=m  TranslationZOffset=0  TranslationZOffsetUnits=m  TranslationThetaOffset=0  TranslationThetaOffsetUnits=deg  RotationMethod=ArbitraryAxis  RotationAngleUnits=rad  RotationStandardAxis=+Z  RotationAngle=1.5707963267948968  RotationArbitraryAxis=[0 1 0]  FollAlignAxisA=+X  BaseAlignAxisA=+Y  FollAlignAxisB=+Y  BaseAlignAxisB=+Z  RotationSequenceAxes=FollowerAxes  RotationSequence=XYX  RotationSequenceAngles=[0 0 0]  RotationSequenceAnglesUnits=deg  RotationMatrix=[1 0 0; 0 1 0; 0 0 1]  BlockFunction=simmechanics.library.frames_transforms.rigid_transform
  Transform15 : sm_lib/Frames and Transforms/Rigid Transform  TranslationMethod=Cartesian  TranslationLengthUnit=mm  TranslationStandardAxis=+Z  TranslationStandardOffset=0  TranslationCartesianOffset=[-119.67899999999999 82.1584 -39.164299999999997]  TranslationROffset=0  TranslationROffsetUnits=m  TranslationZOffset=0  TranslationZOffsetUnits=m  TranslationThetaOffset=0  TranslationThetaOffsetUnits=deg  RotationMethod=ArbitraryAxis  RotationAngleUnits=rad  RotationStandardAxis=+Z  RotationAngle=1.5707963267948968  RotationArbitraryAxis=[0 1 0]  FollAlignAxisA=+X  BaseAlignAxisA=+Y  FollAlignAxisB=+Y  BaseAlignAxisB=+Z  RotationSequenceAxes=FollowerAxes  RotationSequence=XYX  RotationSequenceAngles=[0 0 0]  RotationSequenceAnglesUnits=deg  RotationMatrix=[1 0 0; 0 1 0; 0 0 1]  BlockFunction=simmechanics.library.frames_transforms.rigid_transform
  Transform16 : sm_lib/Frames and Transforms/Rigid Transform  TranslationMethod=Cartesian  TranslationLengthUnit=mm  TranslationStandardAxis=+Z  TranslationStandardOffset=0  TranslationCartesianOffset=[-119.67899999999999 118.61799999999999 -54.614200000000004]  TranslationROffset=0  TranslationROffsetUnits=m  TranslationZOffset=0  TranslationZOffsetUnits=m  TranslationThetaOffset=0  TranslationThetaOffsetUnits=deg  RotationMethod=ArbitraryAxis  RotationAngleUnits=rad  RotationStandardAxis=+Z  RotationAngle=1.5707963267948968  RotationArbitraryAxis=[0 1 0]  FollAlignAxisA=+X  BaseAlignAxisA=+Y  FollAlignAxisB=+Y  BaseAlignAxisB=+Z  RotationSequenceAxes=FollowerAxes  RotationSequence=XYX  RotationSequenceAngles=[0 0 0]  RotationSequenceAnglesUnits=deg  RotationMatrix=[1 0 0; 0 1 0; 0 0 1]  BlockFunction=simmechanics.library.frames_transforms.rigid_transform
  Transform2 : sm_lib/Frames and Transforms/Rigid Transform  TranslationMethod=Cartesian  TranslationLengthUnit=mm  TranslationStandardAxis=+Z  TranslationStandardOffset=0  TranslationCartesianOffset=[-120.379 92.663200000000003 -65.119]  TranslationROffset=0  TranslationROffsetUnits=m  TranslationZOffset=0  TranslationZOffsetUnits=m  TranslationThetaOffset=0  TranslationThetaOffsetUnits=deg  RotationMethod=ArbitraryAxis  RotationAngleUnits=rad  RotationStandardAxis=+Z  RotationAngle=0.4008151858122066  RotationArbitraryAxis=[-1 0 0]  FollAlignAxisA=+X  BaseAlignAxisA=+Y  FollAlignAxisB=+Y  BaseAlignAxisB=+Z  RotationSequenceAxes=FollowerAxes  RotationSequence=XYX  RotationSequenceAngles=[0 0 0]  RotationSequenceAnglesUnits=deg  RotationMatrix=[1 0 0; 0 1 0; 0 0 1]  BlockFunction=simmechanics.library.frames_transforms.rigid_transform
  Transform3 : sm_lib/Frames and Transforms/Rigid Transform  TranslationMethod=Cartesian  TranslationLengthUnit=mm  TranslationStandardAxis=+Z  TranslationStandardOffset=0  TranslationCartesianOffset=[0.72103200000000012 92.663200000000003 -65.119]  TranslationROffset=0  TranslationROffsetUnits=m  TranslationZOffset=0  TranslationZOffsetUnits=m  TranslationThetaOffset=0  TranslationThetaOffsetUnits=deg  RotationMethod=None  RotationAngleUnits=deg  RotationStandardAxis=+Z  RotationAngle=0  RotationArbitraryAxis=[0 0 1]  FollAlignAxisA=+X  BaseAlignAxisA=+Y  FollAlignAxisB=+Y  BaseAlignAxisB=+Z  RotationSequenceAxes=FollowerAxes  RotationSequence=XYX  RotationSequenceAngles=[0 0 0]  RotationSequenceAnglesUnits=deg  RotationMatrix=[1 0 0; 0 1 0; 0 0 1]  BlockFunction=simmechanics.library.frames_transforms.rigid_transform
  Transform4 : sm_lib/Frames and Transforms/Rigid Transform  TranslationMethod=Cartesian  TranslationLengthUnit=mm  TranslationStandardAxis=+Z  TranslationStandardOffset=0  TranslationCartesianOffset=[209.721 92.663200000000003 -65.119]  TranslationROffset=0  TranslationROffsetUnits=m  TranslationZOffset=0  TranslationZOffsetUnits=m  TranslationThetaOffset=0  TranslationThetaOffsetUnits=deg  RotationMethod=ArbitraryAxis  RotationAngleUnits=rad  RotationStandardAxis=+Z  RotationAngle=0.4008151858122066  RotationArbitraryAxis=[-1 0 0]  FollAlignAxisA=+X  BaseAlignAxisA=+Y  FollAlignAxisB=+Y  BaseAlignAxisB=+Z  RotationSequenceAxes=FollowerAxes  RotationSequence=XYX  RotationSequenceAngles=[0 0 0]  RotationSequenceAnglesUnits=deg  RotationMatrix=[1 0 0; 0 1 0; 0 0 1]  BlockFunction=simmechanics.library.frames_transforms.rigid_transform
  Transform5 : sm_lib/Frames and Transforms/Rigid Transform  TranslationMethod=Cartesian  TranslationLengthUnit=mm  TranslationStandardAxis=+Z  TranslationStandardOffset=0  TranslationCartesianOffset=[211.721 66.708399999999997 -75.623800000000003]  TranslationROffset=0  TranslationROffsetUnits=m  TranslationZOffset=0  TranslationZOffsetUnits=m  TranslationThetaOffset=0  TranslationThetaOffsetUnits=deg  RotationMethod=ArbitraryAxis  RotationAngleUnits=rad  RotationStandardAxis=+Z  RotationAngle=2.2403741760322426  RotationArbitraryAxis=[0.61884210013763996 -0.4838066868021465 -0.61884210013763996]  FollAlignAxisA=+X  BaseAlignAxisA=+Y  FollAlignAxisB=+Y  BaseAlignAxisB=+Z  RotationSequenceAxes=FollowerAxes  RotationSequence=XYX  RotationSequenceAngles=[0 0 0]  RotationSequenceAnglesUnits=deg  RotationMatrix=[1 0 0; 0 1 0; 0 0 1]  BlockFunction=simmechanics.library.frames_transforms.rigid_transform
  Transform6 : sm_lib/Frames and Transforms/Rigid Transform  TranslationMethod=Cartesian  TranslationLengthUnit=mm  TranslationStandardAxis=+Z  TranslationStandardOffset=0  TranslationCartesianOffset=[211.721 118.61799999999999 -54.614200000000004]  TranslationROffset=0  TranslationROffsetUnits=m  TranslationZOffset=0  TranslationZOffsetUnits=m  TranslationThetaOffset=0  TranslationThetaOffsetUnits=deg  RotationMethod=ArbitraryAxis  RotationAngleUnits=rad  RotationStandardAxis=+Z  RotationAngle=1.6807030591510466  RotationArbitraryAxis=[0.3143944175699786 -0.89571887353212987 -0.3143944175699786]  FollAlignAxisA=+X  BaseAlignAxisA=+Y  FollAlignAxisB=+Y  BaseAlignAxisB=+Z  RotationSequenceAxes=FollowerAxes  RotationSequence=XYX  RotationSequenceAngles=[0 0 0]  RotationSequenceAnglesUnits=deg  RotationMatrix=[1 0 0; 0 1 0; 0 0 1]  BlockFunction=simmechanics.library.frames_transforms.rigid_transform
  Transform7 : sm_lib/Frames and Transforms/Rigid Transform  TranslationMethod=Cartesian  TranslationLengthUnit=mm  TranslationStandardAxis=+Z  TranslationStandardOffset=0  TranslationCartesianOffset=[211.721 103.16799999999999 -91.073799999999991]  TranslationROffset=0  TranslationROffsetUnits=m  TranslationZOffset=0  TranslationZOffsetUnits=m  TranslationThetaOffset=0  TranslationThetaOffsetUnits=deg  RotationMethod=ArbitraryAxis  RotationAngleUnits=rad  RotationStandardAxis=+Z  RotationAngle=1.9661449904590567  RotationArbitraryAxis=[0.52730076233200707 -0.66626407083690797 -0.52730076233200707]  FollAlignAxisA=+X  BaseAlignAxisA=+Y  FollAlignAxisB=+Y  BaseAlignAxisB=+Z  RotationSequenceAxes=FollowerAxes  RotationSequence=XYX  RotationSequenceAngles=[0 0 0]  RotationSequenceAnglesUnits=deg  RotationMatrix=[1 0 0; 0 1 0; 0 0 1]  BlockFunction=simmechanics.library.frames_transforms.rigid_transform
  Transform8 : sm_lib/Frames and Transforms/Rigid Transform  TranslationMethod=Cartesian  TranslationLengthUnit=mm  TranslationStandardAxis=+Z  TranslationStandardOffset=0  TranslationCartesianOffset=[211.721 82.1584 -39.164299999999997]  TranslationROffset=0  TranslationROffsetUnits=m  TranslationZOffset=0  TranslationZOffsetUnits=m  TranslationThetaOffset=0  TranslationThetaOffsetUnits=deg  RotationMethod=ArbitraryAxis  RotationAngleUnits=rad  RotationStandardAxis=+Z  RotationAngle=1.6229175782530343  RotationArbitraryAxis=[-0.22252615512295251 -0.94919135087314799 0.22252615512295251]  FollAlignAxisA=+X  BaseAlignAxisA=+Y  FollAlignAxisB=+Y  BaseAlignAxisB=+Z  RotationSequenceAxes=FollowerAxes  RotationSequence=XYX  RotationSequenceAngles=[0 0 0]  RotationSequenceAnglesUnits=deg  RotationMatrix=[1 0 0; 0 1 0; 0 0 1]  BlockFunction=simmechanics.library.frames_transforms.rigid_transform
  Transform9 : sm_lib/Frames and Transforms/Rigid Transform  TranslationMethod=Cartesian  TranslationLengthUnit=mm  TranslationStandardAxis=+Z  TranslationStandardOffset=0  TranslationCartesianOffset=[-113.27900000000001 118.61799999999999 -54.614200000000004]  TranslationROffset=0  TranslationROffsetUnits=m  TranslationZOffset=0  TranslationZOffsetUnits=m  TranslationThetaOffset=0  TranslationThetaOffsetUnits=deg  RotationMethod=ArbitraryAxis  RotationAngleUnits=rad  RotationStandardAxis=+Z  RotationAngle=1.6089415653150072  RotationArbitraryAxis=[0.19166392654548026 -0.96256422046652934 -0.19166392654548026]  FollAlignAxisA=+X  BaseAlignAxisA=+Y  FollAlignAxisB=+Y  BaseAlignAxisB=+Z  RotationSequenceAxes=FollowerAxes  RotationSequence=XYX  RotationSequenceAngles=[0 0 0]  RotationSequenceAnglesUnits=deg  RotationMatrix=[1 0 0; 0 1 0; 0 0 1]  BlockFunction=simmechanics.library.frames_transforms.rigid_transform
  Tube_V2H40_1_RIGID : Subsystem
  ecrouM6_1_RIGID : Subsystem
  ecrouM6_2_RIGID : Subsystem
  ecrouM6_3_RIGID : Subsystem
  ecrouM6_4_RIGID : Subsystem
  F1 : PMIOPort  Port=1  Side=Left
  F : PMIOPort  Port=2  Side=Right
  connections:
  Transform/LConn1 -- ReferenceFrame/RConn1 -- Transform1/LConn1 -- Transform10/LConn1 -- Transform11/LConn1 -- Transform12/LConn1 -- Transform13/LConn1 -- Transform14/LConn1 -- Transform15/LConn1 -- Transform16/LConn1 -- Transform2/LConn1 -- Transform3/LConn1 -- Transform4/LConn1 -- Transform5/LConn1 -- Transform6/LConn1 -- Transform7/LConn1 -- Transform8/LConn1 -- Transform9/LConn1
  Transform/RConn1 -- F/RConn1
  Rondelle_M6_1_RIGID/LConn1 -- Transform9/RConn1
  Rondelle_M6_2_RIGID/LConn1 -- Transform10/RConn1
  Rondelle_M6_3_RIGID/LConn1 -- Transform11/RConn1
  Rondelle_M6_4_RIGID/LConn1 -- Transform12/RConn1
  Transform13/RConn1 -- ecrouM6_1_RIGID/LConn1
  Transform14/RConn1 -- ecrouM6_2_RIGID/LConn1
  Transform15/RConn1 -- ecrouM6_3_RIGID/LConn1
  Transform16/RConn1 -- ecrouM6_4_RIGID/LConn1
  Transform1/RConn1 -- F1/RConn1
  Fond_V2H40_1_RIGID/LConn1 -- Transform2/RConn1
  Transform3/RConn1 -- Tube_V2H40_1_RIGID/LConn1
  Nez_V2H40_1_RIGID/LConn1 -- Transform4/RConn1
  Tirant_1_RIGID/LConn1 -- Transform5/RConn1
  Tirant_2_RIGID/LConn1 -- Transform6/RConn1
  Tirant_3_RIGID/LConn1 -- Transform7/RConn1
  Tirant_4_RIGID/LConn1 -- Transform8/RConn1
